simulink model "powerss"  (R2021b)
settings: Solver=VariableStepAuto  StartTime=0.0  StopTime=10.0  RelTol=1e-3
values from neighbouring files (symbols this model uses):
  a = 0.7    [power.m]
  Cd = 0.5    [power.m]
  Cr = 0.004    [power.m]
  D = 1.2    [power.m]
  phi = 2.5    [power.m]
  time = 2    [power.m]
  v = 50    [power.m]
  w = 2000    [power.m]
settings Model: Creator=Madhav R  LastModifiedBy=Madhav R

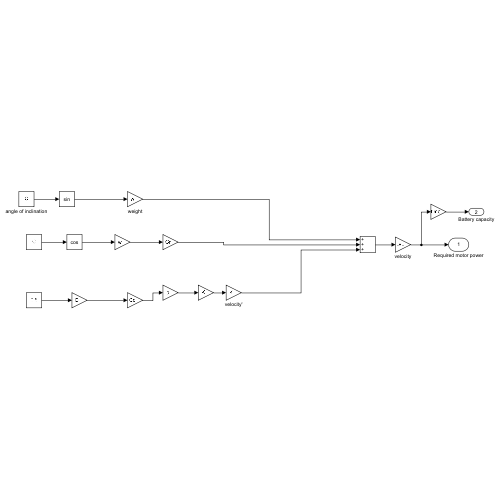
[thumbnail: Simulink's stored preview of the top-level diagram]
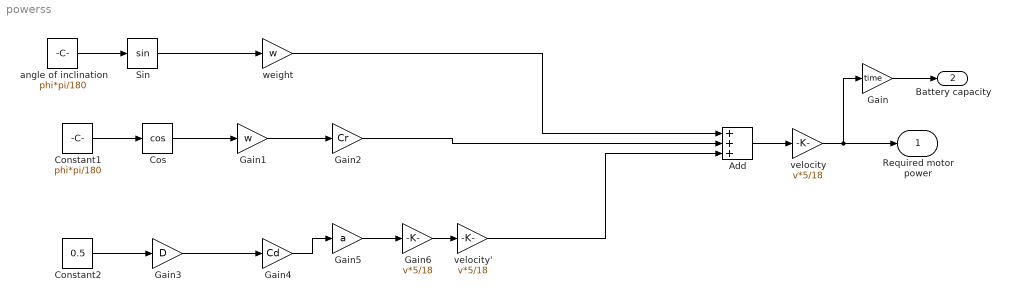
== system powerss ==
  Add : Sum  Inputs=+++
  Constant1 : Constant  Value=phi*pi/180
  Constant2 : Constant  Value=0.5
  Cos : Trigonometry  Operator=cos
  Gain : Gain  Gain=time
  Gain1 : Gain  Gain=w
  Gain2 : Gain  Gain=Cr
  Gain3 : Gain  Gain=D
  Gain4 : Gain  Gain=Cd
  Gain5 : Gain  Gain=a
  Gain6 : Gain  Gain=v*5/18
  Sin : Trigonometry
  angle of inclination : Constant  Value=phi*pi/180
  velocity : Gain  Gain=v*5/18
  velocity' : Gain  Gain=v*5/18
  weight : Gain  Gain=w
  Required motor power : Outport
  Battery capacity : Outport  Port=2
  wires:
  angle of inclination/1 -> Sin/1
  Sin/1 -> weight/1
  Gain1/1 -> Gain2/1
  Constant1/1 -> Cos/1
  Cos/1 -> Gain1/1
  Constant2/1 -> Gain3/1
  Gain3/1 -> Gain4/1
  Gain4/1 -> Gain5/1
  Gain5/1 -> Gain6/1
  Gain6/1 -> velocity'/1
  weight/1 -> Add/1
  Gain2/1 -> Add/2
  velocity'/1 -> Add/3
  Add/1 -> velocity/1
  velocity/1 -> Gain/1, Required motor power/1
  Gain/1 -> Battery capacity/1
